simulink model "gm_uz_mlp_three_layer"  (R2021a)
settings: Solver=FixedStepDiscrete  StartTime=0.0  StopTime=5000  RelTol=1e-3
undefined symbols (not defined in the file or in its folder): nn, nn_data_type_max, numInput, numOut
libraries: hdlsllib x94, simulink x85
(part 4 of 4)

== system gm_uz_mlp_three_layer/uz_mlp_three_layer/LastLayer/parallelOutput/holdValue2 ==
  takeNewValue : Inport  OutDataTypeStr=boolean  PortDimensions=1  SampleTime=1
  data : Inport  Port=2  OutDataTypeStr=fixdt(1, 32, 14)  PortDimensions=1  SampleTime=1
  Delay1 : Delay  DelayLength=1
  Switch : Switch  Criteria=u2 ~= 0
  out : Outport  SampleTime=1
  wires:
  takeNewValue/1 -> Switch/2
  data/1 -> Switch/1
  Delay1/1 -> Switch/3
  Switch/1 -> Delay1/1, out/1

== system gm_uz_mlp_three_layer/uz_mlp_three_layer/LastLayer/parallelOutput/holdValue3 ==
  takeNewValue : Inport  OutDataTypeStr=boolean  PortDimensions=1  SampleTime=1
  data : Inport  Port=2  OutDataTypeStr=fixdt(1, 32, 14)  PortDimensions=1  SampleTime=1
  Delay1 : Delay  DelayLength=1
  Switch : Switch  Criteria=u2 ~= 0
  out : Outport  SampleTime=1
  wires:
  takeNewValue/1 -> Switch/2
  data/1 -> Switch/1
  Delay1/1 -> Switch/3
  Switch/1 -> Delay1/1, out/1

== system gm_uz_mlp_three_layer/uz_mlp_three_layer/LastLayer/parallelOutput/holdValue4 ==
  takeNewValue : Inport  OutDataTypeStr=boolean  PortDimensions=1  SampleTime=1
  data : Inport  Port=2  OutDataTypeStr=fixdt(1, 32, 14)  PortDimensions=1  SampleTime=1
  Delay1 : Delay  DelayLength=1
  Switch : Switch  Criteria=u2 ~= 0
  out : Outport  SampleTime=1
  wires:
  takeNewValue/1 -> Switch/2
  data/1 -> Switch/1
  Delay1/1 -> Switch/3
  Switch/1 -> Delay1/1, out/1

== system gm_uz_mlp_three_layer/uz_mlp_three_layer/LastLayer/parallelOutput/holdValue5 ==
  takeNewValue : Inport  OutDataTypeStr=boolean  PortDimensions=1  SampleTime=1
  data : Inport  Port=2  OutDataTypeStr=fixdt(1, 32, 14)  PortDimensions=1  SampleTime=1
  Delay1 : Delay  DelayLength=1
  Switch : Switch  Criteria=u2 ~= 0
  out : Outport  SampleTime=1
  wires:
  takeNewValue/1 -> Switch/2
  data/1 -> Switch/1
  Delay1/1 -> Switch/3
  Switch/1 -> Delay1/1, out/1

== system gm_uz_mlp_three_layer/uz_mlp_three_layer/LastLayer/parallelOutput/holdValue6 ==
  takeNewValue : Inport  OutDataTypeStr=boolean  PortDimensions=1  SampleTime=1
  data : Inport  Port=2  OutDataTypeStr=fixdt(1, 32, 14)  PortDimensions=1  SampleTime=1
  Delay1 : Delay  DelayLength=1
  Switch : Switch  Criteria=u2 ~= 0
  out : Outport  SampleTime=1
  wires:
  takeNewValue/1 -> Switch/2
  data/1 -> Switch/1
  Delay1/1 -> Switch/3
  Switch/1 -> Delay1/1, out/1

== system gm_uz_mlp_three_layer/uz_mlp_three_layer/LastLayer/parallelOutput/holdValue7 ==
  takeNewValue : Inport  OutDataTypeStr=boolean  PortDimensions=1  SampleTime=1
  data : Inport  Port=2  OutDataTypeStr=fixdt(1, 32, 14)  PortDimensions=1  SampleTime=1
  Delay1 : Delay  DelayLength=1
  Switch : Switch  Criteria=u2 ~= 0
  out : Outport  SampleTime=1
  wires:
  takeNewValue/1 -> Switch/2
  data/1 -> Switch/1
  Delay1/1 -> Switch/3
  Switch/1 -> Delay1/1, out/1

== system gm_uz_mlp_three_layer/uz_mlp_three_layer/reluLayer_4Parallel/StateMachines1/layer_control ==
  ext_enable : Inport  OutDataTypeStr=boolean  PortDimensions=1  SampleTime=1
  mac_ready : Inport  Port=2  OutDataTypeStr=boolean  PortDimensions=1  SampleTime=1
  cnt_finished : Inport  Port=3  OutDataTypeStr=boolean  PortDimensions=1  SampleTime=1
  layer_control : Stateflow chart  TreatAsAtomicUnit=on
  enable_mac : Outport  SampleTime=1
  layer_rdy : Outport  Port=2  SampleTime=1
  cnt_enable : Outport  Port=3  SampleTime=1
  counter_rest : Outport  Port=4  SampleTime=1
  layer_finished : Outport  Port=5  SampleTime=1
  wires:
  layer_control/5(layer_finished) -> layer_finished/1
  layer_control/4(counter_rest) -> counter_rest/1
  layer_control/3(cnt_enable) -> cnt_enable/1
  layer_control/2(layer_rdy) -> layer_rdy/1
  layer_control/1(enable_mac) -> enable_mac/1
  cnt_finished/1 -> layer_control/3(cnt_finished)
  mac_ready/1 -> layer_control/2(mac_ready)
  ext_enable/1 -> layer_control/1(ext_enable)

== system gm_uz_mlp_three_layer/uz_mlp_three_layer/reluLayer_4Parallel/StateMachines1/mac_control ==
  external_enable : Inport  OutDataTypeStr=boolean  PortDimensions=1  SampleTime=1
  counter_finished : Inport  Port=2  OutDataTypeStr=boolean  PortDimensions=1  SampleTime=1
  end_out : Inport  Port=3  OutDataTypeStr=boolean  PortDimensions=1  SampleTime=1
  end_out_delay : Inport  Port=4  OutDataTypeStr=boolean  PortDimensions=1  SampleTime=1
  mac_startOut : Inport  Port=5  OutDataTypeStr=boolean  PortDimensions=1  SampleTime=1
  mac_control : Stateflow chart  TreatAsAtomicUnit=on
  index_counter_enb : Outport  SampleTime=1
  mac_startIn : Outport  Port=2  SampleTime=1
  mac_endIn : Outport  Port=3  SampleTime=1
  mac_validIn : Outport  Port=4  SampleTime=1
  index_counter_rst : Outport  Port=5  SampleTime=1
  write_ram : Outport  Port=6  SampleTime=1
  mac_ready : Outport  Port=7  SampleTime=1
  wires:
  mac_control/7(mac_ready) -> mac_ready/1
  mac_control/6(write_ram) -> write_ram/1
  mac_control/5(index_counter_rst) -> index_counter_rst/1
  mac_control/4(mac_validIn) -> mac_validIn/1
  mac_control/3(mac_endIn) -> mac_endIn/1
  mac_control/2(mac_startIn) -> mac_startIn/1
  mac_control/1(index_counter_enb) -> index_counter_enb/1
  mac_startOut/1 -> mac_control/5(mac_startOut)
  end_out_delay/1 -> mac_control/4(end_out_delay)
  end_out/1 -> mac_control/3(end_out)
  counter_finished/1 -> mac_control/2(counter_finished)
  external_enable/1 -> mac_control/1(external_enable)

== system gm_uz_mlp_three_layer/uz_mlp_three_layer/reluLayer_8Parallel/StateMachines1/layer_control ==
  ext_enable : Inport  OutDataTypeStr=boolean  PortDimensions=1  SampleTime=1
  mac_ready : Inport  Port=2  OutDataTypeStr=boolean  PortDimensions=1  SampleTime=1
  cnt_finished : Inport  Port=3  OutDataTypeStr=boolean  PortDimensions=1  SampleTime=1
  layer_control : Stateflow chart  TreatAsAtomicUnit=on
  enable_mac : Outport  SampleTime=1
  layer_rdy : Outport  Port=2  SampleTime=1
  cnt_enable : Outport  Port=3  SampleTime=1
  counter_rest : Outport  Port=4  SampleTime=1
  layer_finished : Outport  Port=5  SampleTime=1
  wires:
  layer_control/5(layer_finished) -> layer_finished/1
  layer_control/4(counter_rest) -> counter_rest/1
  layer_control/3(cnt_enable) -> cnt_enable/1
  layer_control/2(layer_rdy) -> layer_rdy/1
  layer_control/1(enable_mac) -> enable_mac/1
  cnt_finished/1 -> layer_control/3(cnt_finished)
  mac_ready/1 -> layer_control/2(mac_ready)
  ext_enable/1 -> layer_control/1(ext_enable)

== system gm_uz_mlp_three_layer/uz_mlp_three_layer/reluLayer_8Parallel/StateMachines1/mac_control ==
  external_enable : Inport  OutDataTypeStr=boolean  PortDimensions=1  SampleTime=1
  counter_finished : Inport  Port=2  OutDataTypeStr=boolean  PortDimensions=1  SampleTime=1
  end_out : Inport  Port=3  OutDataTypeStr=boolean  PortDimensions=1  SampleTime=1
  end_out_delay : Inport  Port=4  OutDataTypeStr=boolean  PortDimensions=1  SampleTime=1
  mac_startOut : Inport  Port=5  OutDataTypeStr=boolean  PortDimensions=1  SampleTime=1
  mac_control : Stateflow chart  TreatAsAtomicUnit=on
  index_counter_enb : Outport  SampleTime=1
  mac_startIn : Outport  Port=2  SampleTime=1
  mac_endIn : Outport  Port=3  SampleTime=1
  mac_validIn : Outport  Port=4  SampleTime=1
  index_counter_rst : Outport  Port=5  SampleTime=1
  write_ram : Outport  Port=6  SampleTime=1
  mac_ready : Outport  Port=7  SampleTime=1
  wires:
  mac_control/7(mac_ready) -> mac_ready/1
  mac_control/6(write_ram) -> write_ram/1
  mac_control/5(index_counter_rst) -> index_counter_rst/1
  mac_control/4(mac_validIn) -> mac_validIn/1
  mac_control/3(mac_endIn) -> mac_endIn/1
  mac_control/2(mac_startIn) -> mac_startIn/1
  mac_control/1(index_counter_enb) -> index_counter_enb/1
  mac_startOut/1 -> mac_control/5(mac_startOut)
  end_out_delay/1 -> mac_control/4(end_out_delay)
  end_out/1 -> mac_control/3(end_out)
  counter_finished/1 -> mac_control/2(counter_finished)
  external_enable/1 -> mac_control/1(external_enable)

== system gm_uz_mlp_three_layer/uz_mlp_three_layer/reluLayer_8Parallel1/StateMachines1/layer_control ==
  ext_enable : Inport  OutDataTypeStr=boolean  PortDimensions=1  SampleTime=1
  mac_ready : Inport  Port=2  OutDataTypeStr=boolean  PortDimensions=1  SampleTime=1
  cnt_finished : Inport  Port=3  OutDataTypeStr=boolean  PortDimensions=1  SampleTime=1
  layer_control : Stateflow chart  TreatAsAtomicUnit=on
  enable_mac : Outport  SampleTime=1
  layer_rdy : Outport  Port=2  SampleTime=1
  cnt_enable : Outport  Port=3  SampleTime=1
  counter_rest : Outport  Port=4  SampleTime=1
  layer_finished : Outport  Port=5  SampleTime=1
  wires:
  layer_control/5(layer_finished) -> layer_finished/1
  layer_control/4(counter_rest) -> counter_rest/1
  layer_control/3(cnt_enable) -> cnt_enable/1
  layer_control/2(layer_rdy) -> layer_rdy/1
  layer_control/1(enable_mac) -> enable_mac/1
  cnt_finished/1 -> layer_control/3(cnt_finished)
  mac_ready/1 -> layer_control/2(mac_ready)
  ext_enable/1 -> layer_control/1(ext_enable)

== system gm_uz_mlp_three_layer/uz_mlp_three_layer/reluLayer_8Parallel1/StateMachines1/mac_control ==
  external_enable : Inport  OutDataTypeStr=boolean  PortDimensions=1  SampleTime=1
  counter_finished : Inport  Port=2  OutDataTypeStr=boolean  PortDimensions=1  SampleTime=1
  end_out : Inport  Port=3  OutDataTypeStr=boolean  PortDimensions=1  SampleTime=1
  end_out_delay : Inport  Port=4  OutDataTypeStr=boolean  PortDimensions=1  SampleTime=1
  mac_startOut : Inport  Port=5  OutDataTypeStr=boolean  PortDimensions=1  SampleTime=1
  mac_control : Stateflow chart  TreatAsAtomicUnit=on
  index_counter_enb : Outport  SampleTime=1
  mac_startIn : Outport  Port=2  SampleTime=1
  mac_endIn : Outport  Port=3  SampleTime=1
  mac_validIn : Outport  Port=4  SampleTime=1
  index_counter_rst : Outport  Port=5  SampleTime=1
  write_ram : Outport  Port=6  SampleTime=1
  mac_ready : Outport  Port=7  SampleTime=1
  wires:
  mac_control/7(mac_ready) -> mac_ready/1
  mac_control/6(write_ram) -> write_ram/1
  mac_control/5(index_counter_rst) -> index_counter_rst/1
  mac_control/4(mac_validIn) -> mac_validIn/1
  mac_control/3(mac_endIn) -> mac_endIn/1
  mac_control/2(mac_startIn) -> mac_startIn/1
  mac_control/1(index_counter_enb) -> index_counter_enb/1
  mac_startOut/1 -> mac_control/5(mac_startOut)
  end_out_delay/1 -> mac_control/4(end_out_delay)
  end_out/1 -> mac_control/3(end_out)
  counter_finished/1 -> mac_control/2(counter_finished)
  external_enable/1 -> mac_control/1(external_enable)

== stateflow chart gm_uz_mlp_three_layer/uz_mlp_three_layer/reluLayer_8Parallel/StateMachines1/layer_control/layer_control ==
  settings: executeAtInitialization=1
  state entry_to_entry_state
    layer_rdy=true;
    counter_rest=true; % reset counter for looping through perceptrons of one layer
  state calc_perceptron
    enable_mac=true;
  state idle
    cnt_enable=false;
  state finished2
    layer_finished=false;
  state perceptron_rdy
    cnt_enable=true;
    counter_rest=false;
  state finished
    layer_finished=true;
  state calc_running
    enable_mac=false;
  (default) -> entry_to_entry_state
  finished2 -> entry_to_entry_state
  entry_to_entry_state -> idle : [ext_enable==true]
  idle -> calc_perceptron : [mac_ready==true ]
  calc_perceptron -> calc_running : [mac_ready==false]
  perceptron_rdy -> idle
  finished -> finished2
  calc_running -> perceptron_rdy [order 1] : [mac_ready==true && cnt_finished==false]
  calc_running -> finished [order 2] : [mac_ready==true & cnt_finished==true]
  data: ext_enable input boolean; enable_mac output boolean; mac_ready input boolean; layer_rdy output boolean; cnt_enable output boolean; counter_rest output boolean; cnt_finished input boolean; layer_finished output

== stateflow chart gm_uz_mlp_three_layer/uz_mlp_three_layer/reluLayer_8Parallel/StateMachines1/mac_control/mac_control ==
  settings: executeAtInitialization=1
  state idle_entry
    index_counter_rst=true;
    index_counter_enb=false;
    mac_startIn=false;
    mac_endIn=false;
    mac_validIn=false;
    mac_ready=true;
    write_ram=false;
  state start_counter
    index_counter_rst=false;
    index_counter_enb=true;
    mac_ready=false;
  state write_ram_entry
    write_ram=true;
  state start_mac
    mac_startIn=true;
    mac_validIn=true;
  state accumulate
    mac_startIn=false;
  state mac_stop
    mac_endIn=false;
    mac_validIn=false;
    index_counter_rst=true;
    index_counter_enb=false;
  state mac_finished
    mac_endIn=true;
  (default) -> idle_entry
  idle_entry -> start_counter : [external_enable==true]
  write_ram_entry -> idle_entry
  start_counter -> start_mac
  mac_stop -> write_ram_entry : [end_out_delay==true]
  start_mac -> accumulate : [mac_startOut==true]
  accumulate -> mac_finished : [counter_finished==true]
  mac_finished -> mac_stop : [end_out==true]
  data: index_counter_enb output boolean; mac_startIn output boolean; mac_endIn output boolean; mac_validIn output boolean; index_counter_rst output boolean; external_enable input boolean; counter_finished input boolean; end_out input boolean; end_out_delay input boolean; write_ram output boolean; mac_startOut input boolean; mac_ready output boolean

== stateflow chart gm_uz_mlp_three_layer/uz_mlp_three_layer/reluLayer_8Parallel1/StateMachines1/layer_control/layer_control ==
  settings: executeAtInitialization=1
  state entry_to_entry_state
    layer_rdy=true;
    counter_rest=true; % reset counter for looping through perceptrons of one layer
  state calc_perceptron
    enable_mac=true;
  state idle
    cnt_enable=false;
  state finished2
    layer_finished=false;
  state perceptron_rdy
    cnt_enable=true;
    counter_rest=false;
  state finished
    layer_finished=true;
  state calc_running
    enable_mac=false;
  (default) -> entry_to_entry_state
  finished2 -> entry_to_entry_state
  entry_to_entry_state -> idle : [ext_enable==true]
  idle -> calc_perceptron : [mac_ready==true ]
  calc_perceptron -> calc_running : [mac_ready==false]
  perceptron_rdy -> idle
  finished -> finished2
  calc_running -> perceptron_rdy [order 1] : [mac_ready==true && cnt_finished==false]
  calc_running -> finished [order 2] : [mac_ready==true & cnt_finished==true]
  data: ext_enable input boolean; enable_mac output boolean; mac_ready input boolean; layer_rdy output boolean; cnt_enable output boolean; counter_rest output boolean; cnt_finished input boolean; layer_finished output

== stateflow chart gm_uz_mlp_three_layer/uz_mlp_three_layer/reluLayer_8Parallel1/StateMachines1/mac_control/mac_control ==
  settings: executeAtInitialization=1
  state idle_entry
    index_counter_rst=true;
    index_counter_enb=false;
    mac_startIn=false;
    mac_endIn=false;
    mac_validIn=false;
    mac_ready=true;
    write_ram=false;
  state start_counter
    index_counter_rst=false;
    index_counter_enb=true;
    mac_ready=false;
  state write_ram_entry
    write_ram=true;
  state start_mac
    mac_startIn=true;
    mac_validIn=true;
  state accumulate
    mac_startIn=false;
  state mac_stop
    mac_endIn=false;
    mac_validIn=false;
    index_counter_rst=true;
    index_counter_enb=false;
  state mac_finished
    mac_endIn=true;
  (default) -> idle_entry
  idle_entry -> start_counter : [external_enable==true]
  write_ram_entry -> idle_entry
  start_counter -> start_mac
  mac_stop -> write_ram_entry : [end_out_delay==true]
  start_mac -> accumulate : [mac_startOut==true]
  accumulate -> mac_finished : [counter_finished==true]
  mac_finished -> mac_stop : [end_out==true]
  data: index_counter_enb output boolean; mac_startIn output boolean; mac_endIn output boolean; mac_validIn output boolean; index_counter_rst output boolean; external_enable input boolean; counter_finished input boolean; end_out input boolean; end_out_delay input boolean; write_ram output boolean; mac_startOut input boolean; mac_ready output boolean

== matlab function gm_uz_mlp_three_layer/uz_mlp_three_layer/reluLayer_8Parallel1/MATLAB Function1/MATLAB Function1 ==
  settings: fimath=fimath('RoundingMethod', 'Floor','OverflowAction', 'Wrap','ProductMode', 'FullPrecision', 'SumMode', 'FullPrecision')
  data: readAddr input; y output
function y = fcn(readAddr)

y=uint8(0);
if (readAddr>0 && readAddr <= 8)
    y=uint8(0);
end
if (readAddr>8 && readAddr <= 16)
    y=uint8(1);
end
if (readAddr>16 && readAddr <= 24)
    y=uint8(2);
end
if (readAddr>24 && readAddr <= 32)
    y=uint8(3);
end
if (readAddr>32 && readAddr <= 40)
    y=uint8(4);
end
if (readAddr>40 && readAddr <= 48)
    y=uint8(5);
end
if (readAddr>48 && readAddr <= 56)
    y=uint8(6);
end
if (readAddr>56 && readAddr <= 64)
    y=uint8(7);
end

== matlab function gm_uz_mlp_three_layer/uz_mlp_three_layer/reluLayer_8Parallel/MATLAB Function1/MATLAB Function1 ==
  settings: fimath=fimath('RoundingMethod', 'Floor','OverflowAction', 'Wrap','ProductMode', 'FullPrecision', 'SumMode', 'FullPrecision')
  data: readAddr input; y output
function y = fcn(readAddr)

y=uint8(0);
if (readAddr>0 && readAddr <= 8)
    y=uint8(0);
end
if (readAddr>8 && readAddr <= 16)
    y=uint8(1);
end
if (readAddr>16 && readAddr <= 24)
    y=uint8(2);
end
if (readAddr>24 && readAddr <= 32)
    y=uint8(3);
end
if (readAddr>32 && readAddr <= 40)
    y=uint8(4);
end
if (readAddr>40 && readAddr <= 48)
    y=uint8(5);
end
if (readAddr>48 && readAddr <= 56)
    y=uint8(6);
end
if (readAddr>56 && readAddr <= 64)
    y=uint8(7);
end

== matlab function gm_uz_mlp_three_layer/uz_mlp_three_layer/reluLayer_4Parallel/MATLAB Function/MATLAB Function ==
  settings: fimath=fimath('RoundingMethod', 'Floor','OverflowAction', 'Wrap','ProductMode', 'FullPrecision', 'SumMode', 'FullPrecision')
  data: readAddr input; y output
function y = fcn(readAddr)

y=uint8(0);
if (readAddr>0 && readAddr <= 16)
    y=uint8(0);
end
if (readAddr>16 && readAddr <= 32)
    y=uint8(1);
end
if (readAddr>32 && readAddr <= 48)
    y=uint8(2);
end
if (readAddr>48 && readAddr <= 64)
    y=uint8(3);
end

== stateflow chart gm_uz_mlp_three_layer/uz_mlp_three_layer/LastLayer/StateMachines/layer_control/layer_control ==
  settings: executeAtInitialization=1
  state entry_to_entry_state
    layer_rdy=true;
    counter_rest=true; % reset counter for looping through perceptrons of one layer
  state calc_perceptron
    enable_mac=true;
  state idle
    cnt_enable=false;
  state finished2
    layer_finished=false;
  state perceptron_rdy
    cnt_enable=true;
    counter_rest=false;
  state finished
    layer_finished=true;
  state calc_running
    enable_mac=false;
  (default) -> entry_to_entry_state
  finished2 -> entry_to_entry_state
  entry_to_entry_state -> idle : [ext_enable==true]
  idle -> calc_perceptron : [mac_ready==true ]
  calc_perceptron -> calc_running : [mac_ready==false]
  perceptron_rdy -> idle
  finished -> finished2
  calc_running -> perceptron_rdy [order 1] : [mac_ready==true && cnt_finished==false]
  calc_running -> finished [order 2] : [mac_ready==true & cnt_finished==true]
  data: ext_enable input boolean; enable_mac output boolean; mac_ready input boolean; layer_rdy output boolean; cnt_enable output boolean; counter_rest output boolean; cnt_finished input boolean; layer_finished output

== stateflow chart gm_uz_mlp_three_layer/uz_mlp_three_layer/LastLayer/StateMachines/mac_control/mac_control ==
  settings: executeAtInitialization=1
  state idle_entry
    index_counter_rst=true;
    index_counter_enb=false;
    mac_startIn=false;
    mac_endIn=false;
    mac_validIn=false;
    mac_ready=true;
    write_ram=false;
  state start_counter
    index_counter_rst=false;
    index_counter_enb=true;
    mac_ready=false;
  state write_ram_entry
    write_ram=true;
  state start_mac
    mac_startIn=true;
    mac_validIn=true;
  state accumulate
    mac_startIn=false;
  state mac_stop
    mac_endIn=false;
    mac_validIn=false;
    index_counter_rst=true;
    index_counter_enb=false;
  state mac_finished
    mac_endIn=true;
  (default) -> idle_entry
  idle_entry -> start_counter : [external_enable==true]
  write_ram_entry -> idle_entry
  start_counter -> start_mac
  mac_stop -> write_ram_entry : [end_out_delay==true]
  start_mac -> accumulate : [mac_startOut==true]
  accumulate -> mac_finished : [counter_finished==true]
  mac_finished -> mac_stop : [end_out==true]
  data: index_counter_enb output boolean; mac_startIn output boolean; mac_endIn output boolean; mac_validIn output boolean; index_counter_rst output boolean; external_enable input boolean; counter_finished input boolean; end_out input boolean; end_out_delay input boolean; write_ram output boolean; mac_startOut input boolean; mac_ready output boolean

== stateflow chart gm_uz_mlp_three_layer/uz_mlp_three_layer/reluLayer_4Parallel/StateMachines1/layer_control/layer_control ==
  settings: executeAtInitialization=1
  state entry_to_entry_state
    layer_rdy=true;
    counter_rest=true; % reset counter for looping through perceptrons of one layer
  state calc_perceptron
    enable_mac=true;
  state idle
    cnt_enable=false;
  state finished2
    layer_finished=false;
  state perceptron_rdy
    cnt_enable=true;
    counter_rest=false;
  state finished
    layer_finished=true;
  state calc_running
    enable_mac=false;
  (default) -> entry_to_entry_state
  finished2 -> entry_to_entry_state
  entry_to_entry_state -> idle : [ext_enable==true]
  idle -> calc_perceptron : [mac_ready==true ]
  calc_perceptron -> calc_running : [mac_ready==false]
  perceptron_rdy -> idle
  finished -> finished2
  calc_running -> perceptron_rdy [order 1] : [mac_ready==true && cnt_finished==false]
  calc_running -> finished [order 2] : [mac_ready==true & cnt_finished==true]
  data: ext_enable input boolean; enable_mac output boolean; mac_ready input boolean; layer_rdy output boolean; cnt_enable output boolean; counter_rest output boolean; cnt_finished input boolean; layer_finished output

== stateflow chart gm_uz_mlp_three_layer/uz_mlp_three_layer/reluLayer_4Parallel/StateMachines1/mac_control/mac_control ==
  settings: executeAtInitialization=1
  state idle_entry
    index_counter_rst=true;
    index_counter_enb=false;
    mac_startIn=false;
    mac_endIn=false;
    mac_validIn=false;
    mac_ready=true;
    write_ram=false;
  state start_counter
    index_counter_rst=false;
    index_counter_enb=true;
    mac_ready=false;
  state write_ram_entry
    write_ram=true;
  state start_mac
    mac_startIn=true;
    mac_validIn=true;
  state accumulate
    mac_startIn=false;
  state mac_stop
    mac_endIn=false;
    mac_validIn=false;
    index_counter_rst=true;
    index_counter_enb=false;
  state mac_finished
    mac_endIn=true;
  (default) -> idle_entry
  idle_entry -> start_counter : [external_enable==true]
  write_ram_entry -> idle_entry
  start_counter -> start_mac
  mac_stop -> write_ram_entry : [end_out_delay==true]
  start_mac -> accumulate : [mac_startOut==true]
  accumulate -> mac_finished : [counter_finished==true]
  mac_finished -> mac_stop : [end_out==true]
  data: index_counter_enb output boolean; mac_startIn output boolean; mac_endIn output boolean; mac_validIn output boolean; index_counter_rst output boolean; external_enable input boolean; counter_finished input boolean; end_out input boolean; end_out_delay input boolean; write_ram output boolean; mac_startOut input boolean; mac_ready output boolean
